simulink model "sensor2sensor"  (R2018b)
settings: Solver=FixedStepAuto  StartTime=0.0  StopTime=param.tfinal  FixedStep=param.dt  RelTol=1e-3
values from neighbouring files (symbols this model uses):
  param = quadparam    [quadDyn.m]    (also in quadDynSimple.m; quadSimRunMain.m; quadcomputeFandT.m; quadcomputeMotorSpeed.m)
settings Model: Creator=duho46  LastModifiedBy=duho46

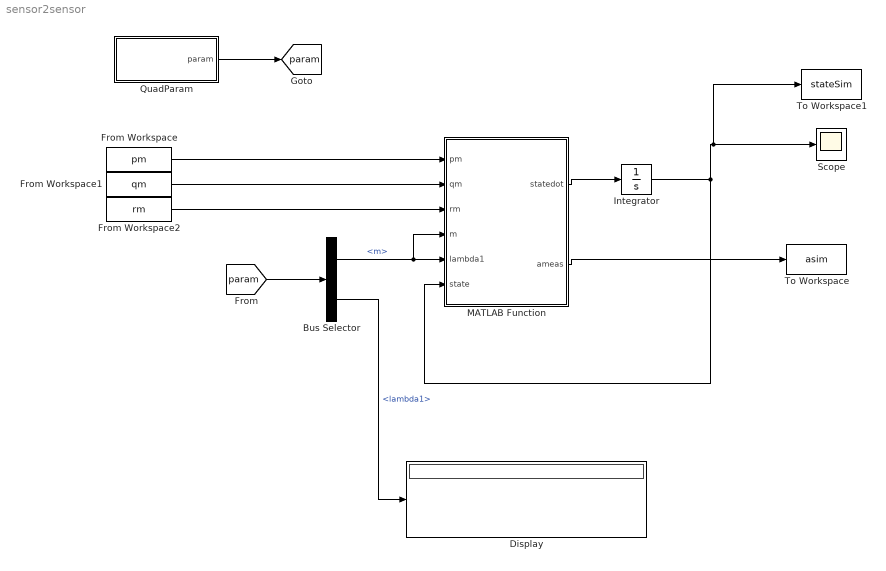
== system sensor2sensor ==
  Bus Selector : BusSelector  OutputSignals=m,lambda1
  Display : Display
  From Workspace : FromWorkspace  VariableName=pm  SampleTime=0
  From Workspace1 : FromWorkspace  VariableName=qm  SampleTime=0
  From Workspace2 : FromWorkspace  VariableName=rm  SampleTime=0
  Integrator : Integrator  InitialCondition=[0 0 0 0]'
  MATLAB Function : MATLAB Function  TreatAsAtomicUnit=on
  QuadParam : Subsystem
  Scope : Scope
  To Workspace : ToWorkspace  VariableName=asim  SampleTime=-1
  To Workspace1 : ToWorkspace  VariableName=stateSim  SampleTime=-1
  tag scope: param=global
  wires:
  QuadParam/1(param) -> [param]
  MATLAB Function/1(statedot) -> Integrator/1
  From Workspace/1 -> MATLAB Function/1(pm)
  From Workspace1/1 -> MATLAB Function/2(qm)
  From Workspace2/1 -> MATLAB Function/3(rm)
  Integrator/1 -> MATLAB Function/6(state), To Workspace1/1, Scope/1
  MATLAB Function/2(ameas) -> To Workspace/1
  [param] -> Bus Selector/1
  Bus Selector/1 -> MATLAB Function/4(m), MATLAB Function/5(lambda1)  "<m>"
  Bus Selector/2 -> Display/1  "<lambda1>"

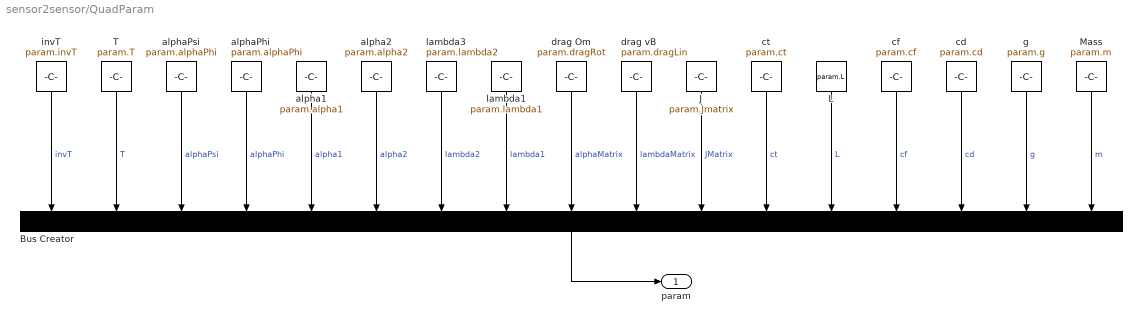
== system sensor2sensor/QuadParam ==
  Bus Creator : BusCreator  Inputs=17
  J : Constant  Value=param.Jmatrix  VectorParams1D=off  OutDataTypeStr=double  SampleTime=-1
  L : Constant  Value=param.L
  Mass : Constant  Value=param.m
  T : Constant  Value=param.T
  "alpha1 " : Constant  Value=param.alpha1
  alpha2 : Constant  Value=param.alpha2
  alphaPhi : Constant  Value=param.alphaPhi
  alphaPsi : Constant  Value=param.alphaPhi
  cd : Constant  Value=param.cd
  cf : Constant  Value=param.cf
  ct : Constant  Value=param.ct
  drag Om : Constant  Value=param.dragRot  VectorParams1D=off
  drag vB : Constant  Value=param.dragLin  VectorParams1D=off
  g : Constant  Value=param.g
  invT : Constant  Value=param.invT
  lambda1 : Constant  Value=param.lambda1
  lambda3 : Constant  Value=param.lambda2
  param : Outport
  wires:
  invT/1 -> Bus Creator/1  "invT"
  T/1 -> Bus Creator/2  "T"
  alphaPsi/1 -> Bus Creator/3  "alphaPsi"
  alphaPhi/1 -> Bus Creator/4  "alphaPhi"
  "alpha1 "/1 -> Bus Creator/5  "alpha1"
  alpha2/1 -> Bus Creator/6  "alpha2"
  lambda3/1 -> Bus Creator/7  "lambda2"
  lambda1/1 -> Bus Creator/8  "lambda1"
  drag Om/1 -> Bus Creator/9  "alphaMatrix"
  drag vB/1 -> Bus Creator/10  "lambdaMatrix"
  J/1 -> Bus Creator/11  "JMatrix"
  ct/1 -> Bus Creator/12  "ct"
  L/1 -> Bus Creator/13  "L"
  cf/1 -> Bus Creator/14  "cf"
  cd/1 -> Bus Creator/15  "cd"
  g/1 -> Bus Creator/16  "g"
  Mass/1 -> Bus Creator/17  "m"
  Bus Creator/1 -> param/1

== matlab function sensor2sensor/MATLAB Function ==
  data: pm input; statedot output; qm input; rm input; m input; lambda1 input; state input; ameas output
function [statedot, ameas] = timeVaryingSystem(pm, qm, rm, m,lambda1, state)

A = [0 rm 0 0;...
    -rm 0 0 0;...
    0 9.81 -lambda1/m 0;...
    -9.81 0 0 -lambda1/m];
% statedot = zeros(4,1);
statedot = A*state + [pm;qm;0;0];
ameas = lambda1/m*[0 0 1 0;0 0 0 1]*state;
